simulink model "SDS_brk_cbc_v1"  (R2018b)
settings: Solver=ode1  StartTime=0.0  StopTime=Inf  FixedStep=0.001  RelTol=1e-3
PostLoadFcn:
  | , if any(exist('dsrtsu_mdlpostloadfcn', 'file') == [2, 3, 6]), try dsrtsu_mdlpostloadfcn('Execute', bdroot); catch fprintf('Error in PostLoadFcn (dsrtsu_mdlpostloadfcn) for model "%s":\n %s\n', bdroot, lasterr); end, end,
libraries: rtican x11, simulink x5
(part 2 of 4)

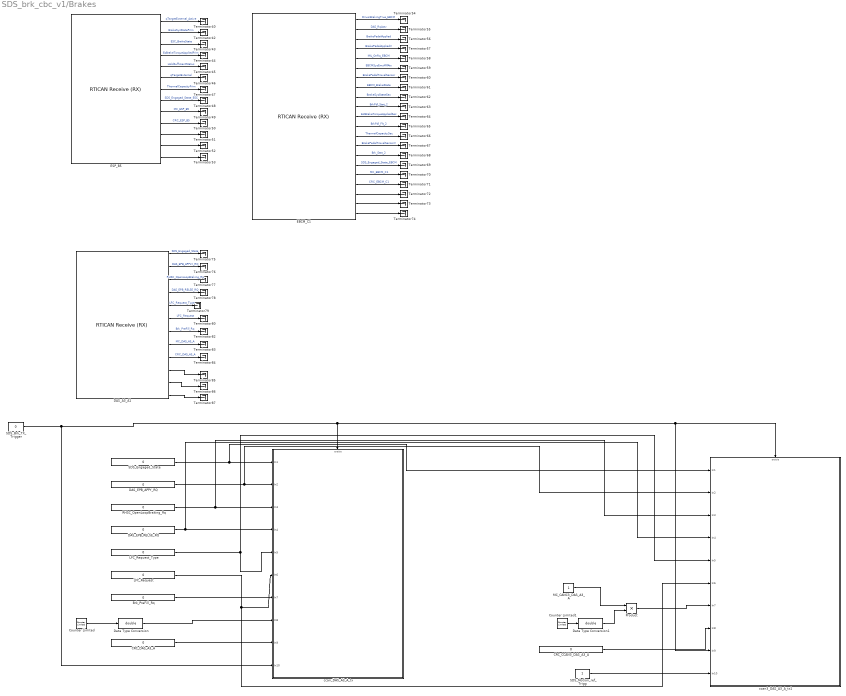
== system SDS_brk_cbc_v1/Brakes ==
  Brk_PreFill_Rq : Constant  Value=0  OutMin=0  OutMax=1  OutDataTypeStr=Inherit: Inherit via back propagation
  CRC_CCAN3_DAS_A3_A : Constant  Value=0  OutMin=0  OutMax=6  OutDataTypeStr=Inherit: Inherit via back propagation
  CRC_DAS_A3_A : Constant  Value=0  OutMin=0  OutMax=6  OutDataTypeStr=Inherit: Inherit via back propagation
  Counter Limited : simulink/Sources/Counter Limited  uplimit=15  tsamp=.01
  Counter Limited1 : simulink/Sources/Counter Limited  uplimit=15  tsamp=.01
  DAS_A3_A1 : rtican/RTICAN Receive (RX)   Reserved1=[]  Reserved2=[]  Reserved3=[]  Reserved4=[]  SfcnMessage=[]  Msg_Struct=[]  BoardTypeNo=[]  BoardNo=[]  ChannelNo=[]  Parameters=[]  DialogFcn=[]  UnitName=[]  Revision=[]  UnitValues=[]  DSProperties=struct('RTI',struct('Version',uint32(5),'BlockType',struct('isSLSource',uint8(1),'isSLSink',uint8(1),'isHWSource',uint8(0),'isHWSink',uint8(0),'isSetup',uint8(0),'isInline',uint8(1),'isNonInline',uint8(0),'isInterrupt',uint8(0),'isChannelwise',uint8(0)),'IOBoardType','RTICAN','UnitType','MESSAGE','Identifier','RX','DialogType','MSVC','BlockSet','RTICAN','SlaveProcessor','CAN'))  RTIBlockInterface=struct('OutputPortsWidth',int32([1 1 1 1 1 1 1 1 1 1 1 1]),'OutputPortsActive',ones(1,12),'OutputPortsName',{{'SDS_Engaged_State','DAS_EPB_APPLY_RQ','RHSC_OpenLoopBraking_Rq','DAS_EPB_RELSE_RQ','LFC_Request_Type','LFC_Request','Brk_PreFill_Rq','MC_DAS_A3_A','CRC_DAS_A3_A',['RX status'],['RX time'],['RX delta time']}},'OutputPortsDataType',{{'SS_DOUBLE','SS_DOUBLE','SS_DOUBLE','SS_DOUBLE','SS_DOUBLE','SS_DOUBLE','SS_DOUBLE','SS_DOUBLE','SS_DOUBLE','SS_DOUBLE','SS_DOUBLE','SS_DOUBLE'}},'OutputPortsLabel',{{'SDS_Engaged_State','DAS_EPB_APPLY_RQ','RHSC_OpenLoopBraking_Rq','DAS_EPB_RELSE_RQ','LFC_Request_Type','LFC_Request','Brk_PreFill_Rq','MC_DAS_A3_A','CRC_DAS_A3_A','','',''}},'OutputPortsLabelMode','ON','InputPortsWidth',int32(0),'InputPortsActive',0,'DialogFcn','rtican_message_interface_gui','BlockDisplay',{{'','center'}},'IconTransparency','on','ParameterTunableNames',{{}},'InitLevel',3,'BlockName',struct('Token',{{'DAS_A3_A'}}),'SampleTime',{{-1}},'TriggerPort',{{'none'}},'EnablePort',{{'none'}})  RTIBlockParameters=struct('BoardTypeNo',{{1,'OFF',[]}},'BoardNo',{{1,'ON',[1 16]}},'ChannelNo',{{1,'ON',[1 2]}},'Parameters',{{struct('DataFileSupport',struct('DataFileSelectedMaster',1,'DataFileSelectedLocal',1,'DataFileName',['c:\intrepidcs\pacifica dbc\e4a_r4_ccan_cr11690_mod.dbc|'],'DataFileDate',{{{['26-Feb-2019 09:24:57']}}},'SelectedFile',['..\..\..\..\..\intrepidcs\pacifica dbc\e4a_r4_ccan_cr11690_mod.dbc']),'Options',struct('StatusSelected',1,'TimeSelected',1,'DeltaTimeSelected',1,'BytePortSelected',0,'MessageLengthSelected',0,'TriggerPort',struct('Selected',0,'TriggerType',0),'UserCoding',struct('Selected',0,'InterfaceFile','UserDecodingFile','FcnName','UserDecodeFcn','InportSelected',0,'InportWidth',1,'OutportSelected',0,'OutportWidth',1),'EnablePortSelected',0,'SignalOnPortnameSelected',1,'UseRXService',0),'Message',struct('MsgOnBlocknameSelected',1,'MsgName','DAS_A3_A','MsgIdFormat',0,'MsgId',499,'MsgLength',8,'NumSignals',9,'SampleTime',-1,'Signal',struct('SgnName',{'SDS_Engaged_State','DAS_EPB_APPLY_RQ','RHSC_OpenLoopBraking_Rq','DAS_EPB_RELSE_RQ','LFC_Request_Type','LFC_Request','Brk_PreFill_Rq','MC_DAS_A3_A','CRC_DAS_A3_A'},'SgnStartBit',{1,3,4,5,6,17,49,52,56},'SgnLength',{2,1,1,1,2,15,1,4,8},'SgnType',{0,0,0,0,0,0,0,0,0},'ModeValue',{-1,-1,-1,-1,-1,-1,-1,-1,-1},'DataType',{0,0,0,0,0,0,0,0,0},'ByteLayout',{0,0,0,0,0,2,0,0,0},'Factor',{1,1,1,1,1,2,1,1,1},'Offset',{0,0,0,0,0,-65534,0,0,0},'SgnComment',{{['SDS Engaged Status']},{['DAS request to apply EPB']},{['Longitudinal Force Control Open Loop Braking Request']},{['DAS request to release EPB']},{['Longitudinal Force Control Request Type']},{''},{['Brakes pre-fill request; True = [1]']},{''},{''}},'SgnUnit',{'','','','','','','','',''},'Min',{0,0,0,0,0,-65534,0,0,0},'Max',{0,0,0,0,0,0,0,15,255},'SLDataType',{'SS_DOUBLE','SS_DOUBLE','SS_DOUBLE','SS_DOUBLE','SS_DOUBLE','SS_DOUBLE','SS_DOUBLE','SS_DOUBLE','SS_DOUBLE'}),'MsgIdNumFormat',0,'MsgComment',{{''}}),'Version',1.2,'general',struct('isFromLib',0)),'OFF',[]}},'GroupId',{{struct('Group',{{'RTICAN'}},'No',1,'Behavior',{{'NAMECHANGE'}},'BlockType',{{'SINK'}},'NameChangeFlag',0),'OFF',[]}},'SFcnRTICANMessage',{{struct('MsgType','RX','SFcnPortType','Scalar','MsgName','DAS_A3_A','MsgIdFormat','STD','MsgId',499,'MsgLength',8,'NumSignals',9,'SampleTime',-1,'Signal',struct('SgnName',{'SDS_Engaged_State','DAS_EPB_APPLY_RQ','RHSC_OpenLoopBraking_Rq','DAS_EPB_RELSE_RQ','LFC_Request_Type','LFC_Request','Brk_PreFill_Rq','MC_DAS_A3_A','CRC_DAS_A3_A'},'SgnStartBit',{1,3,4,5,6,17,49,52,56},'SgnLength',{2,1,1,1,2,15,1,4,8},'SgnType',{'standard','standard','standard','standard','standard','standard','standard','standard','standard'},'ModeValue',{-1,-1,-1,-1,-1,-1,-1,-1,-1},'DataType',{['unsigned int'],['unsigned int'],['unsigned int'],['unsigned int'],['unsigned int'],['unsigned int'],['unsigned int'],['unsigned int'],['unsigned int']},'ByteLayout',{['little endian'],['little endian'],['little endian'],['little endian'],['little endian'],['motorola back.'],['little endian'],['little endian'],['little endian']},'Factor',{1,1,1,1,1,2,1,1,1},'Offset',{0,0,0,0,0,-65534,0,0,0},'SLDataType',{'SS_DOUBLE','SS_DOUBLE','SS_DOUBLE','SS_DOUBLE','SS_DOUBLE','SS_DOUBLE','SS_DOUBLE','SS_DOUBLE','SS_DOUBLE'}),'StatusSelected','yes','TimeSelected','yes','DeltaTimeSelected','yes','BytePortSelected','no','MessageLengthSelected','no','TriggerPort',struct('Selected','no','TriggerType',0),'UserCoding',struct('Selected','no','InterfaceFile','UserDecodingFile','FcnName','UserDecodeFcn','InportSelected','no','InportWidth',1,'OutportSelected','no','OutportWidth',1),'EnablePortSelected','no','UseRXService','no','BoardType','DS1','BoardNo',1,'ControllerNo',2),'OFF',[]}},'TLCFileName',{{'rtican_rx_message','OFF',[]}})  RTISFcnParameters=struct('SFcnRTICANMessage','struct','TLCFileName','char')  RTIBlockParaDefault=struct('BoardTypeNo',4302,'BoardNo',1,'ChannelNo',1,'Parameters',struct('DataFileSupport',struct('DataFileSelectedMaster',0,'DataFileSelectedLocal',0,'DataFileName','','DataFileDate','','SelectedFile',['<no file selected>']),'Options',struct('StatusSelected',1,'TimeSelected',1,'DeltaTimeSelected',1,'BytePortSelected',0,'MessageLengthSelected',0,'TriggerPort',struct('Selected',0,'TriggerType','rising'),'UserCoding',struct('Selected',0,'InterfaceFile','UserDecodingFile','FcnName','UserDecodeFcn','InportSelected',0,'InportWidth',1,'OutportSelected',0,'OutportWidth',1),'EnablePortSelected',0,'SignalOnPortnameSelected',1,'UseRXService',0),'Message',struct('MsgOnBlocknameSelected',0,'MsgName',['RX Message'],'MsgIdFormat',0,'MsgId',100,'MsgLength',8,'NumSignals',1,'SampleTime',-1,'Signal',struct('SgnName',['RX signal'],'SgnStartBit',0,'SgnLength',8,'SgnType',0,'ModeValue',-1,'DataType',0,'SLDataType','SS_DOUBLE','ByteLayout',0,'Factor',1,'Offset',0,'Min',0,'Max',255,'SgnComment',{{}},'SgnUnit',''),'MsgIdNumFormat',0,'MsgComment',{{''}}),'Version',1.2,'general',struct('isFromLib',1)),'GroupId',struct('Group',{{'RTICAN'}},'No',1,'Behavior',{{'NAMECHANGE'}},'BlockType',{{'SINK'}},'NameChangeFlag',0),'SFcnRTICANMessage',struct('MsgType','RX','MsgName',['RX Message'],'MsgIdFormat','STD','MsgId',100,'MsgLength',8,'NumSignals',1,'SampleTime',-1,'Signal',struct('SgnName',['RX signal'],'SgnStartBit',0,'SgnLength',8,'SgnType','standard','ModeValue',-1,'DataType',['unsigned int'],'ByteLayout',['little endian'],'SLDataType','SS_DOUBLE','Factor',1,'Offset',0),'StatusSelected','yes','TimeSelected','yes','DeltaTimeSelected','yes','BytePortSelected','no','MessageLengthSelected','no','EnablePortSelected','no','UserCoding',struct('Selected','no','InterfaceFile','UserDecodingFile','FcnName','UserDecodeFcn','InportSelected','no','InportWidth',1,'OutportSelected','no','OutportWidth',1),'TriggerPort',struct('Selected','no','TriggerType','rising'),'UseRXService','no','BoardType','DS4302','BoardNo',1,'ControllerNo',1,'SFcnPortType','Scalar'),'TLCFileName','rtican_rx_message')
      settings: AttributesFormatString=Group Id: RTICAN1\n  SourceProductName=dSPACE RTI CAN Blockset
  DAS_EPB_APPY_RQ : Constant  Value=0  OutMin=0  OutMax=1  OutDataTypeStr=Inherit: Inherit via back propagation
  DAS_EPB_RELSE_RQ : Constant  Value=0  OutMin=0  OutMax=1  OutDataTypeStr=Inherit: Inherit via back propagation
  Data Type Conversion : DataTypeConversion  OutDataTypeStr=double
  Data Type Conversion1 : DataTypeConversion  OutDataTypeStr=double
  EBCM_C1 : rtican/RTICAN Receive (RX)   Reserved1=[]  Reserved2=[]  Reserved3=[]  Reserved4=[]  SfcnMessage=[]  Msg_Struct=[]  BoardTypeNo=[]  BoardNo=[]  ChannelNo=[]  Parameters=[]  DialogFcn=[]  UnitName=[]  Revision=[]  UnitValues=[]  DSProperties=struct('RTI',struct('Version',uint32(5),'BlockType',struct('isSLSource',uint8(1),'isSLSink',uint8(1),'isHWSource',uint8(0),'isHWSink',uint8(0),'isSetup',uint8(0),'isInline',uint8(1),'isNonInline',uint8(0),'isInterrupt',uint8(0),'isChannelwise',uint8(0)),'IOBoardType','RTICAN','UnitType','MESSAGE','Identifier','RX','DialogType','MSVC','BlockSet','RTICAN','SlaveProcessor','CAN'))  RTIBlockInterface=struct('OutputPortsWidth',int32([1 1 1 1 1 1 1 1 1 1 1 1 1 1 1 1 1 1 1 1 1]),'OutputPortsActive',ones(1,21),'OutputPortsName',{{'DriverBrakingTrue_EBCM','DAS_RqActv','BrakePedalApplied','BrakePedalAppliedV','MIL_OnRq_EBCM','EBCMSysEmsMlfAtv','BrakePedalTravelSensor','EBCM_BrakeState','BrakeSysStateSec','BrkPdl_Stat_2','EstBrakeTorqueAppliedSec','BrkPdl_Flt_2','ThermalCapacitySec','BrakePedalTravelSensorV','Brk_Stat_2','SDS_Engaged_State_EBCM','MC_EBCM_C1','CRC_EBCM_C1',['RX status'],['RX time'],['RX delta time']}},'OutputPortsDataType',{{'SS_DOUBLE','SS_DOUBLE','SS_DOUBLE','SS_DOUBLE','SS_DOUBLE','SS_DOUBLE','SS_DOUBLE','SS_DOUBLE','SS_DOUBLE','SS_DOUBLE','SS_DOUBLE','SS_DOUBLE','SS_DOUBLE','SS_DOUBLE','SS_DOUBLE','SS_DOUBLE','SS_DOUBLE','SS_DOUBLE','SS_DOUBLE','SS_DOUBLE','SS_DOUBLE'}},'OutputPortsLabel',{{'DriverBrakingTrue_EBCM','DAS_RqActv','BrakePedalApplied','BrakePedalAppliedV','MIL_OnRq_EBCM','EBCMSysEmsMlfAtv','BrakePedalTravelSensor','EBCM_BrakeState','BrakeSysStateSec','BrkPdl_Stat_2','EstBrakeTorqueAppliedSec','BrkPdl_Flt_2','ThermalCapacitySec','BrakePedalTravelSensorV','Brk_Stat_2','SDS_Engaged_State_EBCM','MC_EBCM_C1','CRC_EBCM_C1','','',''}},'OutputPortsLabelMode','ON','InputPortsWidth',int32(0),'InputPortsActive',0,'DialogFcn','rtican_message_interface_gui','BlockDisplay',{{'','center'}},'IconTransparency','on','ParameterTunableNames',{{}},'InitLevel',3,'BlockName',struct('Token',{{'EBCM_C1'}}),'SampleTime',{{0}},'TriggerPort',{{'none'}},'EnablePort',{{'none'}})  RTIBlockParameters=struct('BoardTypeNo',{{1,'OFF',[]}},'BoardNo',{{1,'ON',[1 16]}},'ChannelNo',{{1,'ON',[1 2]}},'Parameters',{{struct('DataFileSupport',struct('DataFileSelectedMaster',1,'DataFileSelectedLocal',1,'DataFileName',['c:\intrepidcs\pacifica dbc\e4a_r4_ccan_cr11690_mod.dbc|'],'DataFileDate',{{{['26-Feb-2019 09:25:05']}}},'SelectedFile',['..\..\..\..\..\intrepidcs\pacifica dbc\e4a_r4_ccan_cr11690_mod.dbc']),'Options',struct('StatusSelected',1,'TimeSelected',1,'DeltaTimeSelected',1,'BytePortSelected',0,'MessageLengthSelected',0,'TriggerPort',struct('Selected',0,'TriggerType',0),'UserCoding',struct('Selected',0,'InterfaceFile','UserDecodingFile','FcnName','UserDecodeFcn','InportSelected',0,'InportWidth',1,'OutportSelected',0,'OutportWidth',1),'EnablePortSelected',0,'SignalOnPortnameSelected',1,'UseRXService',0),'Message',struct('MsgOnBlocknameSelected',1,'MsgName','EBCM_C1','MsgIdFormat',0,'MsgId',653,'MsgLength',8,'NumSignals',18,'SampleTime',0,'Signal',struct('SgnName',{'DriverBrakingTrue_EBCM','DAS_RqActv','BrakePedalApplied','BrakePedalAppliedV','MIL_OnRq_EBCM','EBCMSysEmsMlfAtv','BrakePedalTravelSensor','EBCM_BrakeState','BrakeSysStateSec','BrkPdl_Stat_2','EstBrakeTorqueAppliedSec','BrkPdl_Flt_2','ThermalCapacitySec','BrakePedalTravelSensorV','Brk_Stat_2','SDS_Engaged_State_EBCM','MC_EBCM_C1','CRC_EBCM_C1'},'SgnStartBit',{0,1,4,5,6,7,8,16,19,22,24,31,40,46,48,50,52,56},'SgnLength',{1,3,1,1,1,1,8,3,3,2,15,1,6,1,2,2,4,8},'SgnType',{0,0,0,0,0,0,0,0,0,0,0,0,0,0,0,0,0,0},'ModeValue',{-1,-1,-1,-1,-1,-1,-1,-1,-1,-1,-1,-1,-1,-1,-1,-1,-1,-1},'DataType',{0,0,0,0,0,0,0,0,0,0,0,0,0,0,0,0,0,0},'ByteLayout',{0,0,0,0,0,0,0,0,0,0,2,0,0,0,0,0,0,0},'Factor',{1,1,1,1,1,1,0.4,1,1,1,2,1,1.5873,1,1,1,1,1},'Offset',{0,0,0,0,0,0,0,0,0,0,-65534,0,0,0,0,0,0,0},'SgnComment',{{['Driver operates the brake pedal; Pressed = [1]']},{['DAS request active']},{['driver operates the brake pedal']},{['Validity bit']},{['MIL on request from the EBCM']},{['EBCM emissions related malfunction active']},{['Brake pedal travel sensor 0-100% (0 = upstop)']},{['EBCM Brake State']},{['EBCM Brake State from Secondary actuator']},{['Brake pedal state']},{''},{['Brake pedal fault is active; True = [1]']},{''},{['Brake pedal travel sensor valid (1 = valid data)']},{['Brake state']},{['SDS Engaged Status']},{['Message counter']},{['CRC-checksum byte 1 to 7 according to SAE J1850']}},'SgnUnit',{'','','','','','','%','','','','Nm','','%','','','','',''},'Min',{0,0,0,0,0,0,0,0,0,0,-65534,0,0,0,0,0,0,0},'Max',{0,0,0,0,0,0,100,0,0,0,0,0,100,0,0,0,15,0},'SLDataType',{'SS_DOUBLE','SS_DOUBLE','SS_DOUBLE','SS_DOUBLE','SS_DOUBLE','SS_DOUBLE','SS_DOUBLE','SS_DOUBLE','SS_DOUBLE','SS_DOUBLE','SS_DOUBLE','SS_DOUBLE','SS_DOUBLE','SS_DOUBLE','SS_DOUBLE','SS_DOUBLE','SS_DOUBLE','SS_DOUBLE'}),'MsgIdNumFormat',0,'MsgComment',{{''}}),'Version',1.2,'general',struct('isFromLib',0)),'OFF',[]}},'GroupId',{{struct('Group',{{'RTICAN'}},'No',1,'Behavior',{{'NAMECHANGE'}},'BlockType',{{'SINK'}},'NameChangeFlag',0),'OFF',[]}},'SFcnRTICANMessage',{{struct('MsgType','RX','SFcnPortType','Scalar','MsgName','EBCM_C1','MsgIdFormat','STD','MsgId',653,'MsgLength',8,'NumSignals',18,'SampleTime',0,'Signal',struct('SgnName',{'DriverBrakingTrue_EBCM','DAS_RqActv','BrakePedalApplied','BrakePedalAppliedV','MIL_OnRq_EBCM','EBCMSysEmsMlfAtv','BrakePedalTravelSensor','EBCM_BrakeState','BrakeSysStateSec','BrkPdl_Stat_2','EstBrakeTorqueAppliedSec','BrkPdl_Flt_2','ThermalCapacitySec','BrakePedalTravelSensorV','Brk_Stat_2','SDS_Engaged_State_EBCM','MC_EBCM_C1','CRC_EBCM_C1'},'SgnStartBit',{0,1,4,5,6,7,8,16,19,22,24,31,40,46,48,50,52,56},'SgnLength',{1,3,1,1,1,1,8,3,3,2,15,1,6,1,2,2,4,8},'SgnType',{'standard','standard','standard','standard','standard','standard','standard','standard','standard','standard','standard','standard','standard','standard','standard','standard','standard','standard'},'ModeValue',{-1,-1,-1,-1,-1,-1,-1,-1,-1,-1,-1,-1,-1,-1,-1,-1,-1,-1},'DataType',{['unsigned int'],['unsigned int'],['unsigned int'],['unsigned int'],['unsigned int'],['unsigned int'],['unsigned int'],['unsigned int'],['unsigned int'],['unsigned int'],['unsigned int'],['unsigned int'],['unsigned int'],['unsigned int'],['unsigned int'],['unsigned int'],['unsigned int'],['unsigned int']},'ByteLayout',{['little endian'],['little endian'],['little endian'],['little endian'],['little endian'],['little endian'],['little endian'],['little endian'],['little endian'],['little endian'],['motorola back.'],['little endian'],['little endian'],['little endian'],['little endian'],['little endian'],['little endian'],['little endian']},'Factor',{1,1,1,1,1,1,0.4,1,1,1,2,1,1.5873,1,1,1,1,1},'Offset',{0,0,0,0,0,0,0,0,0,0,-65534,0,0,0,0,0,0,0},'SLDataType',{'SS_DOUBLE','SS_DOUBLE','SS_DOUBLE','SS_DOUBLE','SS_DOUBLE','SS_DOUBLE','SS_DOUBLE','SS_DOUBLE','SS_DOUBLE','SS_DOUBLE','SS_DOUBLE','SS_DOUBLE','SS_DOUBLE','SS_DOUBLE','SS_DOUBLE','SS_DOUBLE','SS_DOUBLE','SS_DOUBLE'}),'StatusSelected','yes','TimeSelected','yes','DeltaTimeSelected','yes','BytePortSelected','no','MessageLengthSelected','no','TriggerPort',struct('Selected','no','TriggerType',0),'UserCoding',struct('Selected','no','InterfaceFile','UserDecodingFile','FcnName','UserDecodeFcn','InportSelected','no','InportWidth',1,'OutportSelected','no','OutportWidth',1),'EnablePortSelected','no','UseRXService','no','BoardType','DS1','BoardNo',1,'ControllerNo',1),'OFF',[]}},'TLCFileName',{{'rtican_rx_message','OFF',[]}})  RTISFcnParameters=struct('SFcnRTICANMessage','struct','TLCFileName','char')  RTIBlockParaDefault=struct('BoardTypeNo',4302,'BoardNo',1,'ChannelNo',1,'Parameters',struct('DataFileSupport',struct('DataFileSelectedMaster',0,'DataFileSelectedLocal',0,'DataFileName','','DataFileDate','','SelectedFile',['<no file selected>']),'Options',struct('StatusSelected',1,'TimeSelected',1,'DeltaTimeSelected',1,'BytePortSelected',0,'MessageLengthSelected',0,'TriggerPort',struct('Selected',0,'TriggerType','rising'),'UserCoding',struct('Selected',0,'InterfaceFile','UserDecodingFile','FcnName','UserDecodeFcn','InportSelected',0,'InportWidth',1,'OutportSelected',0,'OutportWidth',1),'EnablePortSelected',0,'SignalOnPortnameSelected',1,'UseRXService',0),'Message',struct('MsgOnBlocknameSelected',0,'MsgName',['RX Message'],'MsgIdFormat',0,'MsgId',100,'MsgLength',8,'NumSignals',1,'SampleTime',-1,'Signal',struct('SgnName',['RX signal'],'SgnStartBit',0,'SgnLength',8,'SgnType',0,'ModeValue',-1,'DataType',0,'SLDataType','SS_DOUBLE','ByteLayout',0,'Factor',1,'Offset',0,'Min',0,'Max',255,'SgnComment',{{}},'SgnUnit',''),'MsgIdNumFormat',0,'MsgComment',{{''}}),'Version',1.2,'general',struct('isFromLib',1)),'GroupId',struct('Group',{{'RTICAN'}},'No',1,'Behavior',{{'NAMECHANGE'}},'BlockType',{{'SINK'}},'NameChangeFlag',0),'SFcnRTICANMessage',struct('MsgType','RX','MsgName',['RX Message'],'MsgIdFormat','STD','MsgId',100,'MsgLength',8,'NumSignals',1,'SampleTime',-1,'Signal',struct('SgnName',['RX signal'],'SgnStartBit',0,'SgnLength',8,'SgnType','standard','ModeValue',-1,'DataType',['unsigned int'],'ByteLayout',['little endian'],'SLDataType','SS_DOUBLE','Factor',1,'Offset',0),'StatusSelected','yes','TimeSelected','yes','DeltaTimeSelected','yes','BytePortSelected','no','MessageLengthSelected','no','EnablePortSelected','no','UserCoding',struct('Selected','no','InterfaceFile','UserDecodingFile','FcnName','UserDecodeFcn','InportSelected','no','InportWidth',1,'OutportSelected','no','OutportWidth',1),'TriggerPort',struct('Selected','no','TriggerType','rising'),'UseRXService','no','BoardType','DS4302','BoardNo',1,'ControllerNo',1,'SFcnPortType','Scalar'),'TLCFileName','rtican_rx_message')
      settings: AttributesFormatString=Group Id: RTICAN1\n  SourceProductName=dSPACE RTI CAN Blockset
  ESP_B5 : rtican/RTICAN Receive (RX)   Reserved1=[]  Reserved2=[]  Reserved3=[]  Reserved4=[]  SfcnMessage=[]  Msg_Struct=[]  BoardTypeNo=[]  BoardNo=[]  ChannelNo=[]  Parameters=[]  DialogFcn=[]  UnitName=[]  Revision=[]  UnitValues=[]  DSProperties=struct('RTI',struct('Version',uint32(5),'BlockType',struct('isSLSource',uint8(1),'isSLSink',uint8(1),'isHWSource',uint8(0),'isHWSink',uint8(0),'isSetup',uint8(0),'isInline',uint8(1),'isNonInline',uint8(0),'isInterrupt',uint8(0),'isChannelwise',uint8(0)),'IOBoardType','RTICAN','UnitType','MESSAGE','Identifier','RX','DialogType','MSVC','BlockSet','RTICAN','SlaveProcessor','CAN'))  RTIBlockInterface=struct('OutputPortsWidth',int32([1 1 1 1 1 1 1 1 1 1 1 1 1]),'OutputPortsActive',ones(1,13),'OutputPortsName',{{'qTargetExternal_Active','BrakeSysStatePrim','ESC_BrakeState','EsBrakeTorqueAppliedPrim','HoldSufficientStatus','qTargetExternal','ThermalCapacityPrim','SDS_Engaged_State_ESC','MC_ESP_B5','CRC_ESP_B5',['RX status'],['RX time'],['RX delta time']}},'OutputPortsDataType',{{'SS_DOUBLE','SS_DOUBLE','SS_DOUBLE','SS_DOUBLE','SS_DOUBLE','SS_DOUBLE','SS_DOUBLE','SS_DOUBLE','SS_DOUBLE','SS_DOUBLE','SS_DOUBLE','SS_DOUBLE','SS_DOUBLE'}},'OutputPortsLabel',{{'qTargetExternal_Active','BrakeSysStatePrim','ESC_BrakeState','EsBrakeTorqueAppliedPrim','HoldSufficientStatus','qTargetExternal','ThermalCapacityPrim','SDS_Engaged_State_ESC','MC_ESP_B5','CRC_ESP_B5','','',''}},'OutputPortsLabelMode','ON','InputPortsWidth',int32(0),'InputPortsActive',0,'DialogFcn','rtican_message_interface_gui','BlockDisplay',{{'','center'}},'IconTransparency','on','ParameterTunableNames',{{}},'InitLevel',3,'BlockName',struct('Token',{{'ESP_B5'}}),'SampleTime',{{0}},'TriggerPort',{{'none'}},'EnablePort',{{'none'}})  RTIBlockParameters=struct('BoardTypeNo',{{1,'OFF',[]}},'BoardNo',{{1,'ON',[1 16]}},'ChannelNo',{{1,'ON',[1 2]}},'Parameters',{{struct('DataFileSupport',struct('DataFileSelectedMaster',1,'DataFileSelectedLocal',1,'DataFileName',['c:\intrepidcs\pacifica dbc\e4a_r4_ccan_cr11690_mod.dbc|'],'DataFileDate',{{{['26-Feb-2019 09:25:05']}}},'SelectedFile',['..\..\..\..\..\intrepidcs\pacifica dbc\e4a_r4_ccan_cr11690_mod.dbc']),'Options',struct('StatusSelected',1,'TimeSelected',1,'DeltaTimeSelected',1,'BytePortSelected',0,'MessageLengthSelected',0,'TriggerPort',struct('Selected',0,'TriggerType',0),'UserCoding',struct('Selected',0,'InterfaceFile','UserDecodingFile','FcnName','UserDecodeFcn','InportSelected',0,'InportWidth',1,'OutportSelected',0,'OutportWidth',1),'EnablePortSelected',0,'SignalOnPortnameSelected',1,'UseRXService',0),'Message',struct('MsgOnBlocknameSelected',1,'MsgName','ESP_B5','MsgIdFormat',0,'MsgId',682,'MsgLength',8,'NumSignals',10,'SampleTime',0,'Signal',struct('SgnName',{'qTargetExternal_Active','BrakeSysStatePrim','ESC_BrakeState','EsBrakeTorqueAppliedPrim','HoldSufficientStatus','qTargetExternal','ThermalCapacityPrim','SDS_Engaged_State_ESC','MC_ESP_B5','CRC_ESP_B5'},'SgnStartBit',{0,2,5,24,31,40,42,50,52,56},'SgnLength',{2,3,3,15,1,16,6,2,4,8},'SgnType',{0,0,0,0,0,0,0,0,0,0},'ModeValue',{-1,-1,-1,-1,-1,-1,-1,-1,-1,-1},'DataType',{0,0,0,0,0,0,0,0,0,0},'ByteLayout',{0,0,0,2,0,2,0,0,0,0},'Factor',{1,1,1,2,1,2^-7,1.5873,1,1,1},'Offset',{0,0,0,-65534,0,-252,0,0,0,0},'SgnComment',{{['Activates the external brake volume flow request when equal to 1']},{['Brake System State from Primary actuator']},{['ESC Brake State']},{''},{['1 � Indicates ESC has sufficient torque, for RHSC to command release of park brake or move out of park. ']},{['Target volume flow speed of the brake system to be applied by iBooster for EBR.']},{''},{['SDS Engaged Status']},{['Message counter']},{['CRC-checksum byte 1 to 7 according to SAE J1850']}},'SgnUnit',{'','','','Nm','','ml/sec','%','','',''},'Min',{0,0,0,-65534,0,-252,0,0,0,0},'Max',{0,0,0,0,0,252,99.9999,0,15,0},'SLDataType',{'SS_DOUBLE','SS_DOUBLE','SS_DOUBLE','SS_DOUBLE','SS_DOUBLE','SS_DOUBLE','SS_DOUBLE','SS_DOUBLE','SS_DOUBLE','SS_DOUBLE'}),'MsgIdNumFormat',0,'MsgComment',{{''}}),'Version',1.2,'general',struct('isFromLib',0)),'OFF',[]}},'GroupId',{{struct('Group',{{'RTICAN'}},'No',1,'Behavior',{{'NAMECHANGE'}},'BlockType',{{'SINK'}},'NameChangeFlag',0),'OFF',[]}},'SFcnRTICANMessage',{{struct('MsgType','RX','SFcnPortType','Scalar','MsgName','ESP_B5','MsgIdFormat','STD','MsgId',682,'MsgLength',8,'NumSignals',10,'SampleTime',0,'Signal',struct('SgnName',{'qTargetExternal_Active','BrakeSysStatePrim','ESC_BrakeState','EsBrakeTorqueAppliedPrim','HoldSufficientStatus','qTargetExternal','ThermalCapacityPrim','SDS_Engaged_State_ESC','MC_ESP_B5','CRC_ESP_B5'},'SgnStartBit',{0,2,5,24,31,40,42,50,52,56},'SgnLength',{2,3,3,15,1,16,6,2,4,8},'SgnType',{'standard','standard','standard','standard','standard','standard','standard','standard','standard','standard'},'ModeValue',{-1,-1,-1,-1,-1,-1,-1,-1,-1,-1},'DataType',{['unsigned int'],['unsigned int'],['unsigned int'],['unsigned int'],['unsigned int'],['unsigned int'],['unsigned int'],['unsigned int'],['unsigned int'],['unsigned int']},'ByteLayout',{['little endian'],['little endian'],['little endian'],['motorola back.'],['little endian'],['motorola back.'],['little endian'],['little endian'],['little endian'],['little endian']},'Factor',{1,1,1,2,1,2^-7,1.5873,1,1,1},'Offset',{0,0,0,-65534,0,-252,0,0,0,0},'SLDataType',{'SS_DOUBLE','SS_DOUBLE','SS_DOUBLE','SS_DOUBLE','SS_DOUBLE','SS_DOUBLE','SS_DOUBLE','SS_DOUBLE','SS_DOUBLE','SS_DOUBLE'}),'StatusSelected','yes','TimeSelected','yes','DeltaTimeSelected','yes','BytePortSelected','no','MessageLengthSelected','no','TriggerPort',struct('Selected','no','TriggerType',0),'UserCoding',struct('Selected','no','InterfaceFile','UserDecodingFile','FcnName','UserDecodeFcn','InportSelected','no','InportWidth',1,'OutportSelected','no','OutportWidth',1),'EnablePortSelected','no','UseRXService','no','BoardType','DS1','BoardNo',1,'ControllerNo',1),'OFF',[]}},'TLCFileName',{{'rtican_rx_message','OFF',[]}})  RTISFcnParameters=struct('SFcnRTICANMessage','struct','TLCFileName','char')  RTIBlockParaDefault=struct('BoardTypeNo',4302,'BoardNo',1,'ChannelNo',1,'Parameters',struct('DataFileSupport',struct('DataFileSelectedMaster',0,'DataFileSelectedLocal',0,'DataFileName','','DataFileDate','','SelectedFile',['<no file selected>']),'Options',struct('StatusSelected',1,'TimeSelected',1,'DeltaTimeSelected',1,'BytePortSelected',0,'MessageLengthSelected',0,'TriggerPort',struct('Selected',0,'TriggerType','rising'),'UserCoding',struct('Selected',0,'InterfaceFile','UserDecodingFile','FcnName','UserDecodeFcn','InportSelected',0,'InportWidth',1,'OutportSelected',0,'OutportWidth',1),'EnablePortSelected',0,'SignalOnPortnameSelected',1,'UseRXService',0),'Message',struct('MsgOnBlocknameSelected',0,'MsgName',['RX Message'],'MsgIdFormat',0,'MsgId',100,'MsgLength',8,'NumSignals',1,'SampleTime',-1,'Signal',struct('SgnName',['RX signal'],'SgnStartBit',0,'SgnLength',8,'SgnType',0,'ModeValue',-1,'DataType',0,'SLDataType','SS_DOUBLE','ByteLayout',0,'Factor',1,'Offset',0,'Min',0,'Max',255,'SgnComment',{{}},'SgnUnit',''),'MsgIdNumFormat',0,'MsgComment',{{''}}),'Version',1.2,'general',struct('isFromLib',1)),'GroupId',struct('Group',{{'RTICAN'}},'No',1,'Behavior',{{'NAMECHANGE'}},'BlockType',{{'SINK'}},'NameChangeFlag',0),'SFcnRTICANMessage',struct('MsgType','RX','MsgName',['RX Message'],'MsgIdFormat','STD','MsgId',100,'MsgLength',8,'NumSignals',1,'SampleTime',-1,'Signal',struct('SgnName',['RX signal'],'SgnStartBit',0,'SgnLength',8,'SgnType','standard','ModeValue',-1,'DataType',['unsigned int'],'ByteLayout',['little endian'],'SLDataType','SS_DOUBLE','Factor',1,'Offset',0),'StatusSelected','yes','TimeSelected','yes','DeltaTimeSelected','yes','BytePortSelected','no','MessageLengthSelected','no','EnablePortSelected','no','UserCoding',struct('Selected','no','InterfaceFile','UserDecodingFile','FcnName','UserDecodeFcn','InportSelected','no','InportWidth',1,'OutportSelected','no','OutportWidth',1),'TriggerPort',struct('Selected','no','TriggerType','rising'),'UseRXService','no','BoardType','DS4302','BoardNo',1,'ControllerNo',1,'SFcnPortType','Scalar'),'TLCFileName','rtican_rx_message')
      settings: AttributesFormatString=Group Id: RTICAN1\n  SourceProductName=dSPACE RTI CAN Blockset
  LFC_Request : Constant  Value=0  OutMin=-10000  OutMax=0  OutDataTypeStr=Inherit: Inherit via back propagation
  LFC_Request_Type : Constant  Value=0  OutMin=0  OutMax=6  OutDataTypeStr=Inherit: Inherit via back propagation
  MC_CANC3_DAS_A3_A : Constant
  Product : Product
  RHSC_OpenLoopBraking_Rq : Constant  Value=0  OutMin=0  OutMax=1  OutDataTypeStr=Inherit: Inherit via back propagation
  SDS_Brk_TX_Trigger : Constant  Value=0  OutDataTypeStr=Inherit: Inherit via back propagation
  SDS_Engaged_State : Constant  Value=0  OutMin=0  OutMax=1  OutDataTypeStr=double
  SDS_Motion_ref_Trigg : Constant  OutDataTypeStr=Inherit: Inherit via back propagation
  Terminator{40,42..80,82..87} (46 alike) : Terminator
  ccan3_DAS_A3_A_tx1 : Subsystem
  ccan_DAS_A3_A_tx : Subsystem
  wires:
  EBCM_C1/2 -> Terminator55/1  "DAS_RqActv"
  EBCM_C1/3 -> Terminator56/1  "BrakePedalApplied"
  EBCM_C1/6 -> Terminator59/1  "EBCMSysEmsMlfAtv"
  DAS_A3_A1/12 -> Terminator87/1
  EBCM_C1/19 -> Terminator72/1
  EBCM_C1/10 -> Terminator63/1  "BrkPdl_Stat_2"
  EBCM_C1/8 -> Terminator61/1  "EBCM_BrakeState"
  DAS_A3_A1/11 -> Terminator86/1
  EBCM_C1/20 -> Terminator73/1
  ESP_B5/13 -> Terminator53/1
  ESP_B5/9 -> Terminator49/1  "MC_ESP_B5"
  DAS_A3_A1/10 -> Terminator85/1
  EBCM_C1/9 -> Terminator62/1  "BrakeSysStateSec"
  ESP_B5/4 -> Terminator44/1  "EsBrakeTorqueAppliedPrim"
  ESP_B5/6 -> Terminator46/1  "qTargetExternal"
  EBCM_C1/1 -> Terminator54/1  "DriverBrakingTrue_EBCM"
  ESP_B5/10 -> Terminator50/1  "CRC_ESP_B5"
  EBCM_C1/17 -> Terminator70/1  "MC_EBCM_C1"
  EBCM_C1/15 -> Terminator68/1  "Brk_Stat_2"
  EBCM_C1/13 -> Terminator66/1  "ThermalCapacitySec"
  ESP_B5/7 -> Terminator47/1  "ThermalCapacityPrim"
  ESP_B5/2 -> Terminator42/1  "BrakeSysStatePrim"
  EBCM_C1/5 -> Terminator58/1  "MIL_OnRq_EBCM"
  EBCM_C1/21 -> Terminator74/1
  ESP_B5/12 -> Terminator52/1
  RHSC_OpenLoopBraking_Rq/1 -> ccan3_DAS_A3_A_tx1/3(In3), ccan_DAS_A3_A_tx/3(In3)
  EBCM_C1/12 -> Terminator65/1  "BrkPdl_Flt_2"
  DAS_EPB_APPY_RQ/1 -> ccan3_DAS_A3_A_tx1/2(In2), ccan_DAS_A3_A_tx/2(In2)
  EBCM_C1/18 -> Terminator71/1  "CRC_EBCM_C1"
  EBCM_C1/7 -> Terminator60/1  "BrakePedalTravelSensor"
  LFC_Request_Type/1 -> ccan3_DAS_A3_A_tx1/5(In5), ccan_DAS_A3_A_tx/5(In5)
  ESP_B5/5 -> Terminator45/1  "HoldSufficientStatus"
  EBCM_C1/4 -> Terminator57/1  "BrakePedalAppliedV"
  ESP_B5/8 -> Terminator48/1  "SDS_Engaged_State_ESC"
  EBCM_C1/14 -> Terminator67/1  "BrakePedalTravelSensorV"
  ESP_B5/11 -> Terminator51/1
  LFC_Request/1 -> ccan3_DAS_A3_A_tx1/6(In6), ccan_DAS_A3_A_tx/6(In6)
  Brk_PreFill_Rq/1 -> ccan_DAS_A3_A_tx/7(In7)
  SDS_Engaged_State/1 -> ccan3_DAS_A3_A_tx1/1(In1), ccan_DAS_A3_A_tx/1(In1)
  ESP_B5/1 -> Terminator40/1  "qTargetExternal_Active"
  EBCM_C1/11 -> Terminator64/1  "EstBrakeTorqueAppliedSec"
  EBCM_C1/16 -> Terminator69/1  "SDS_Engaged_State_EBCM"
  ESP_B5/3 -> Terminator43/1  "ESC_BrakeState"
  DAS_EPB_RELSE_RQ/1 -> ccan3_DAS_A3_A_tx1/4(In4), ccan_DAS_A3_A_tx/4(In4)
  CRC_DAS_A3_A/1 -> ccan_DAS_A3_A_tx/9(In9)
  Data Type Conversion/1 -> ccan_DAS_A3_A_tx/8(In8)
  Counter Limited/1 -> Data Type Conversion/1
  Counter Limited1/1 -> Data Type Conversion1/1
  DAS_A3_A1/1 -> Terminator75/1  "SDS_Engaged_State"
  DAS_A3_A1/2 -> Terminator76/1  "DAS_EPB_APPLY_RQ"
  DAS_A3_A1/3 -> Terminator77/1  "RHSC_OpenLoopBraking_Rq"
  DAS_A3_A1/4 -> Terminator78/1  "DAS_EPB_RELSE_RQ"
  DAS_A3_A1/5 -> Terminator79/1  "LFC_Request_Type"
  DAS_A3_A1/6 -> Terminator80/1  "LFC_Request"
  DAS_A3_A1/9 -> Terminator84/1  "CRC_DAS_A3_A"
  DAS_A3_A1/8 -> Terminator83/1  "MC_DAS_A3_A"
  DAS_A3_A1/7 -> Terminator82/1  "Brk_PreFill_Rq"
  CRC_CCAN3_DAS_A3_A/1 -> ccan3_DAS_A3_A_tx1/8(In8)
  Product/1 -> ccan3_DAS_A3_A_tx1/7(In7)
  Data Type Conversion1/1 -> Product/2
  MC_CANC3_DAS_A3_A/1 -> Product/1
  SDS_Motion_ref_Trigg/1 -> ccan3_DAS_A3_A_tx1/10(In10)
  SDS_Brk_TX_Trigger/1 -> ccan_DAS_A3_A_tx/10(In10), ccan3_DAS_A3_A_tx1/9(In9), ccan3_DAS_A3_A_tx1/Enable, ccan_DAS_A3_A_tx/Enable
